simulink model "zad1_sim"  (R2025a)
settings: Solver=VariableStepAuto  StartTime=0.0  StopTime=10.0  RelTol=1e-3
values from neighbouring files (symbols this model uses):
  A = [0, 1, 0, 0, 0, 0 ... (first row only)    [zad1.m]
  B = zeros(6,1)    [zad1.m]
  C = [1, 0, 0, 0, 0, 0 ... (first row only)    [zad1.m]
  D = [0; 0; 0]    [zad1.m]
  h = 42    [zad1.m]
  k1 = 54.7    [zad1.m]
  k2 = 303.6    [zad1.m]
  m1 = 14000    [zad1.m]
  m2 = 450.28    [zad1.m]
  m3 = 200    [zad1.m]
  X0 = [0; 67; 0; 0; 0; 0]    [zad1.m]
settings Model: Creator=Dejmian  LastModifiedBy=Dejmian

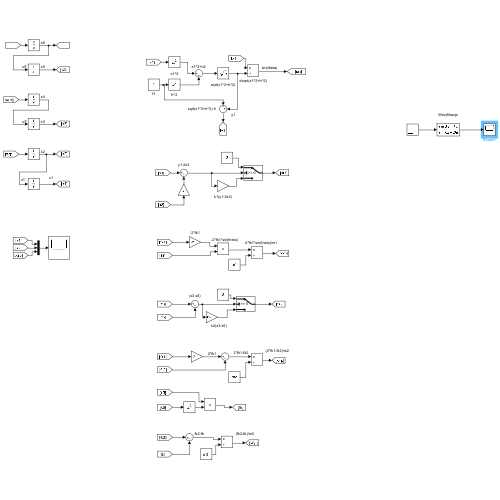
[thumbnail: Simulink's stored preview of the top-level diagram]
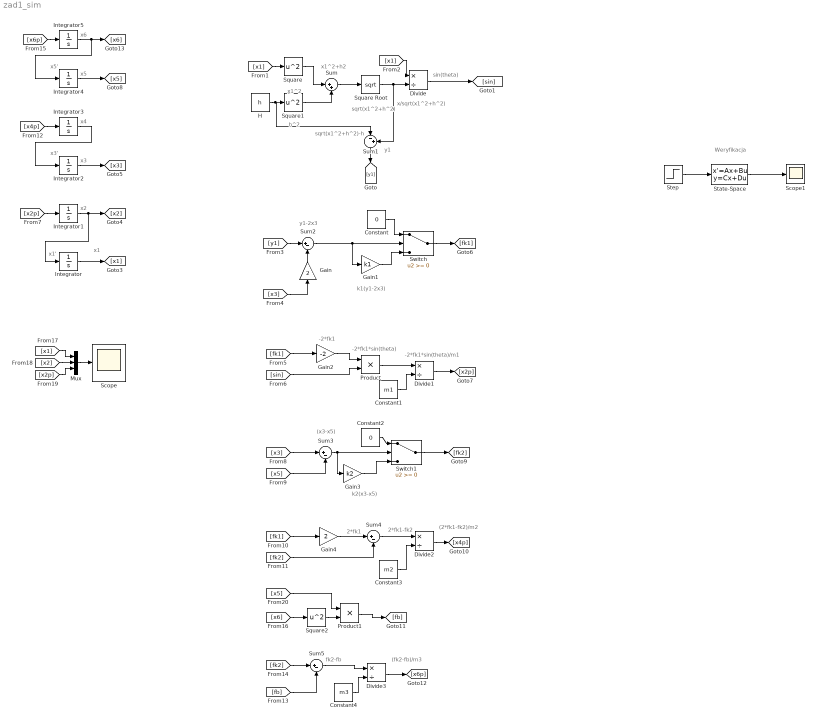
== system zad1_sim ==
  note: Weryfikacja
  note: (fk2-fb)/m3
  note: fk2-fb
  note: (2*fk1-fk2)/m2
  note: 2*fk1-fk2
  note: 2*fk1
  note: k2(x3-x5)
  note: (x3-x5)
  note: -2*fk1*sin(theta)/m1
  note: -2*fk1*sin(theta)
  note: -2*fk1
  note: k1(y1-2x3)
  note: y1-2x3
  note: x4
  note: x3'
  note: x3
  note: x2
  note: x1'
  note: y1
  note: sin(theta)
  note: sqrt(x1^2+h^2)-h
  note: x/sqrt(x1^2+h^2)
  note: sqrt(x1^2+h^2)
  note: x1^2+h2
  note: h^2
  note: x1^2
  note: x1
  note: x6
  note: x5'
  note: x5
  Constant : Constant  Value=0
  Constant1 : Constant  Value=m1
  Constant2 : Constant  Value=0
  Constant3 : Constant  Value=m2
  Constant4 : Constant  Value=m3
  Divide{,1..3} (4 alike) : Product  Inputs=*/
  Gain : Gain  Gain=2
  Gain1 : Gain  Gain=k1
  Gain2 : Gain  Gain=-2
  Gain3 : Gain  Gain=k2
  Gain4 : Gain  Gain=2
  H : Constant  Value=h
  Integrator{,2..5} (5 alike) : Integrator
  Integrator1 : Integrator  InitialCondition=67
  Mux : Mux  Inputs=3
  Product : Product
  Product1 : Product
  Scope : Scope
      settings: ActiveDisplayYMinimum=-83.749999999999915  ActiveDisplayYMaximum=753.74999999999932
  Scope1 : Scope
      settings: ActiveDisplayYMinimum=-83.749999999999915  ActiveDisplayYMaximum=753.74999999999932
  Square : Math  Operator=square
  Square Root : Sqrt
  Square1 : Math  Operator=square
  Square2 : Math  Operator=square
  State-Space : StateSpace  A=A  B=B  C=C  D=D  InitialCondition=X0
  Step : Step  SampleTime=0
  Sum : Sum  Inputs=|++
  Sum1 : Sum  Inputs=|-+
  Sum{2..5} (4 alike) : Sum  Inputs=|+-
  Switch : Switch  SaturateOnIntegerOverflow=off  InputSameDT=off
  Switch1 : Switch  SaturateOnIntegerOverflow=off  InputSameDT=off
  wires:
  H/1 -> Sum1/1, Square1/1
  Square/1 -> Sum/1
  Square1/1 -> Sum/2
  Sum/1 -> Square Root/1
  Square Root/1 -> Sum1/2, Divide/2
  Integrator1/1 -> [x2], Integrator/1
  Sum1/1 -> [y1]
  Divide/1 -> [sin]
  Integrator/1 -> [x1]
  [x1] -> Square/1
  [x1] -> Divide/1
  Integrator3/1 -> Integrator2/1
  Integrator2/1 -> [x3]
  [y1] -> Sum2/1
  Gain/1 -> Sum2/2
  [x3] -> Gain/1
  Sum2/1 -> Gain1/1, Switch/2
  Switch/1 -> [fk1]
  [fk1] -> Gain2/1
  Gain2/1 -> Product/1
  [sin] -> Product/2
  Product/1 -> Divide1/1
  Constant1/1 -> Divide1/2
  Divide1/1 -> [x2p]
  [x2p] -> Integrator1/1
  Integrator5/1 -> [x6], Integrator4/1
  Integrator4/1 -> [x5]
  [x3] -> Sum3/1
  [x5] -> Sum3/2
  Sum3/1 -> Gain3/1, Switch1/2
  Switch1/1 -> [fk2]
  [fk1] -> Gain4/1
  Gain4/1 -> Sum4/1
  [fk2] -> Sum4/2
  Sum4/1 -> Divide2/1
  Constant3/1 -> Divide2/2
  Divide2/1 -> [x4p]
  [x4p] -> Integrator3/1
  [fk2] -> Sum5/1
  [fb] -> Sum5/2
  Sum5/1 -> Divide3/1
  Constant4/1 -> Divide3/2
  Divide3/1 -> [x6p]
  [x6p] -> Integrator5/1
  [x6] -> Square2/1
  Mux/1 -> Scope/1
  [x1] -> Mux/1
  [x2] -> Mux/2
  [x2p] -> Mux/3
  Gain1/1 -> Switch/3
  Constant/1 -> Switch/1
  Gain3/1 -> Switch1/3
  Constant2/1 -> Switch1/1
  State-Space/1 -> Scope1/1
  Step/1 -> State-Space/1
  Square2/1 -> Product1/2
  [x5] -> Product1/1
  Product1/1 -> [fb]
